simulink model "intent_estimator"  (R2024b)
settings: Solver=FixedStepAuto  StartTime=0.0  StopTime=10.0  RelTol=1e-3
settings Model: Creator=lukec  LastModifiedBy=lukec
settings OptimizationCC: DefaultParameterBehavior=Inlined  EnhancedBackFolding=on  PassReuseOutputArgsAs=Individual arguments  ZeroExternalMemoryAtStartup=off  ZeroInternalMemoryAtStartup=off  OptimizeBlockOrder=speed  DifferentSizesBufferReuse=on  OptimizationCustomize=off  EfficientTunableParamExpr=on
settings DebuggingCC: ParameterTunabilityLossMsg=error
settings HardwareCC: ProdBitPerPointer=32  ProdBitPerSizeT=32  ProdBitPerPtrDiffT=32  ProdLargestAtomicInteger=Long  ProdLargestAtomicFloat=Double  ProdWordSize=32  ProdHWDeviceType=ARM Compatible->ARM Cortex-M
settings SFSimCC: MATLABDynamicMemAlloc=off
settings RTWCC: Description=Embedded Coder  SystemTargetFile=ert.tlc  GenCodeOnly=on  PackageGeneratedCodeAndArtifacts=on  TemplateMakefile=ert_default_tmf  Toolchain=CMake  TargetLang=C++  HalideCodeGeneration=on
settings CodeAppCC: ForceParamTrailComments=on  IgnoreCustomStorageClasses=off  MaxIdLength=255  OperatorAnnotations=on  SimulinkDataObjDesc=on  SFDataObjDesc=on  InsertBlockDesc=on
settings ERTTargetCC: TargetLangStandard=C++17 (ISO)  CodeInterfacePackaging=C++ class  RootIOFormat=Structure reference  ERTCustomFileTemplate=example_file_process.tlc  ArrayContainerType=std::array

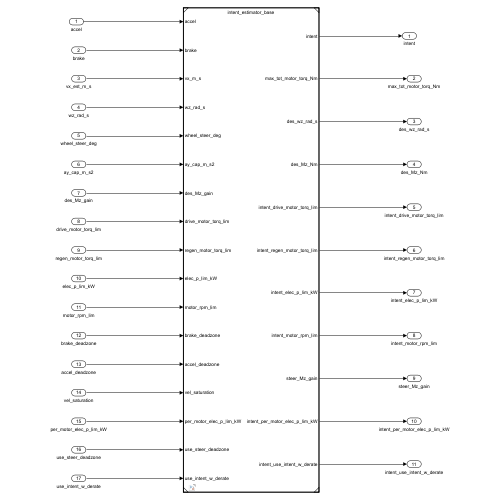
[thumbnail: Simulink's stored preview of the top-level diagram]
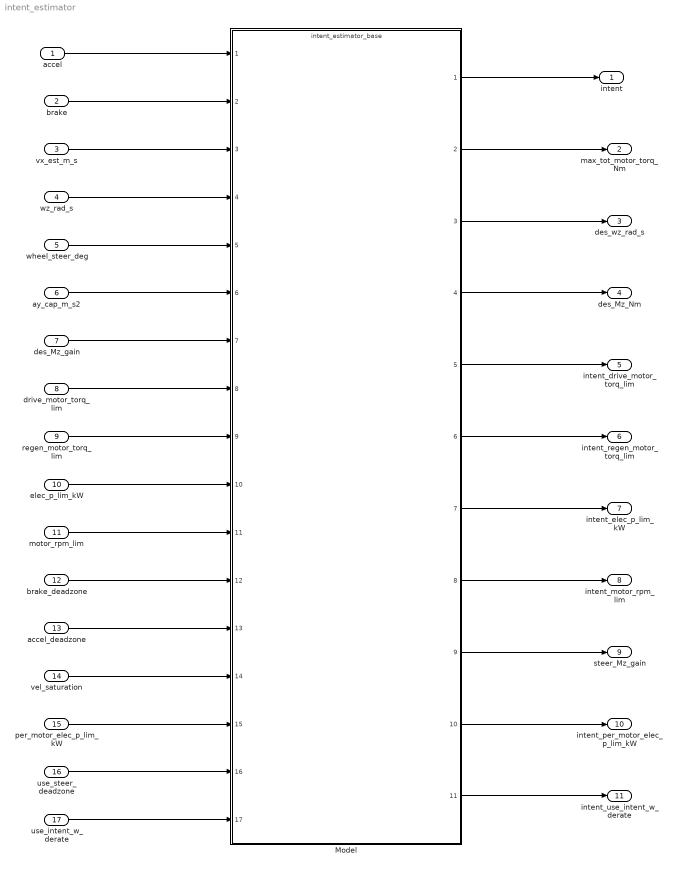
== system intent_estimator ==
  accel : Inport
  brake : Inport  Port=2
  vx_est_m_s : Inport  Port=3
  wz_rad_s : Inport  Port=4
  wheel_steer_deg : Inport  Port=5
  ay_cap_m_s2 : Inport  Port=6
  des_Mz_gain : Inport  Port=7
  drive_motor_torq_lim : Inport  Port=8
  regen_motor_torq_lim : Inport  Port=9
  elec_p_lim_kW : Inport  Port=10
  motor_rpm_lim : Inport  Port=11
  brake_deadzone : Inport  Port=12
  accel_deadzone : Inport  Port=13
  vel_saturation : Inport  Port=14
  per_motor_elec_p_lim_kW : Inport  Port=15
  use_steer_deadzone : Inport  Port=16
  use_intent_w_derate : Inport  Port=17
  Model : ModelReference  ModelNameDialog=intent_estimator_base.slx  SimulationMode=Normal  ModelReferenceVersion=1.19
  intent : Outport
  max_tot_motor_torq_Nm : Outport  Port=2
  des_wz_rad_s : Outport  Port=3
  des_Mz_Nm : Outport  Port=4
  intent_drive_motor_torq_lim : Outport  Port=5
  intent_regen_motor_torq_lim : Outport  Port=6
  intent_elec_p_lim_kW : Outport  Port=7
  intent_motor_rpm_lim : Outport  Port=8
  steer_Mz_gain : Outport  Port=9
  intent_per_motor_elec_p_lim_kW : Outport  Port=10
  intent_use_intent_w_derate : Outport  Port=11
  wires:
  brake/1 -> Model/2
  accel/1 -> Model/1
  vx_est_m_s/1 -> Model/3
  wheel_steer_deg/1 -> Model/5
  ay_cap_m_s2/1 -> Model/6
  wz_rad_s/1 -> Model/4
  drive_motor_torq_lim/1 -> Model/8
  des_Mz_gain/1 -> Model/7
  regen_motor_torq_lim/1 -> Model/9
  motor_rpm_lim/1 -> Model/11
  brake_deadzone/1 -> Model/12
  elec_p_lim_kW/1 -> Model/10
  accel_deadzone/1 -> Model/13
  Model/1 -> intent/1
  Model/2 -> max_tot_motor_torq_Nm/1
  Model/3 -> des_wz_rad_s/1
  Model/4 -> des_Mz_Nm/1
  Model/5 -> intent_drive_motor_torq_lim/1
  Model/6 -> intent_regen_motor_torq_lim/1
  Model/7 -> intent_elec_p_lim_kW/1
  Model/8 -> intent_motor_rpm_lim/1
  vel_saturation/1 -> Model/14
  Model/9 -> steer_Mz_gain/1
  Model/10 -> intent_per_motor_elec_p_lim_kW/1
  per_motor_elec_p_lim_kW/1 -> Model/15
  use_steer_deadzone/1 -> Model/16
  use_intent_w_derate/1 -> Model/17
  Model/11 -> intent_use_intent_w_derate/1
